simulink model "trial2"  (R2020a)
settings: Solver=VariableStepAuto  StartTime=0.0  StopTime=10.0  RelTol=1e-3
settings Model: Creator="mukesh  thota"  LastModifiedBy="mukesh  thota"

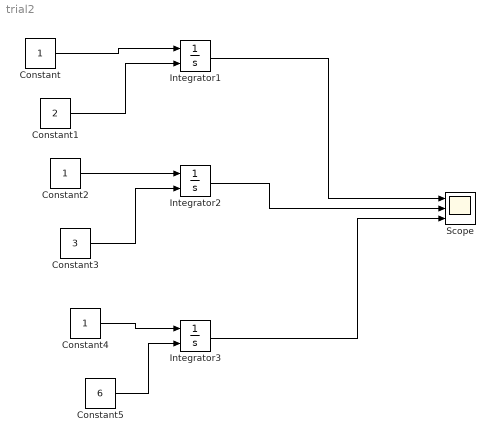
== system trial2 ==
  Constant : Constant
  Constant1 : Constant  Value=2
  Constant2 : Constant
  Constant3 : Constant  Value=3
  Constant4 : Constant
  Constant5 : Constant  Value=6
  Integrator1 : Integrator  InitialConditionSource=external
  Integrator2 : Integrator  InitialConditionSource=external
  Integrator3 : Integrator  InitialConditionSource=external
  Scope : Scope  NumInputPorts=3
  wires:
  Constant/1 -> Integrator1/1
  Constant1/1 -> Integrator1/2
  Constant2/1 -> Integrator2/1
  Constant3/1 -> Integrator2/2
  Constant4/1 -> Integrator3/1
  Constant5/1 -> Integrator3/2
  Integrator1/1 -> Scope/1
  Integrator2/1 -> Scope/2
  Integrator3/1 -> Scope/3
